simulink model "AION_IDS_SPEEDGOAT"  (R2021a)
settings: configuration reference "AION_IDS_Speedgoat" (kept outside this file)
undefined symbols (not defined in the file): ADCU_SCU_CYCLE_TIME, AutoTrqWhlReq_test, BeamReq_test, BodyCtrlReq_test, BrakeReq_test, C, CONTROL_CYCLE_TIME, GearLvlReq_test, GearLvlReqVD_test, HornRingReq_test, LatCtrlReq_test, LngCtrlReq_test, SCU_ADCU_CYCLE_TIME, SteerAngReq_test, SteerWhlTorqReq_test, TurnLightReq_test
libraries: canmsglib x21, speedgoatlib_IO612 x8, simulink x1
(part 2 of 2)

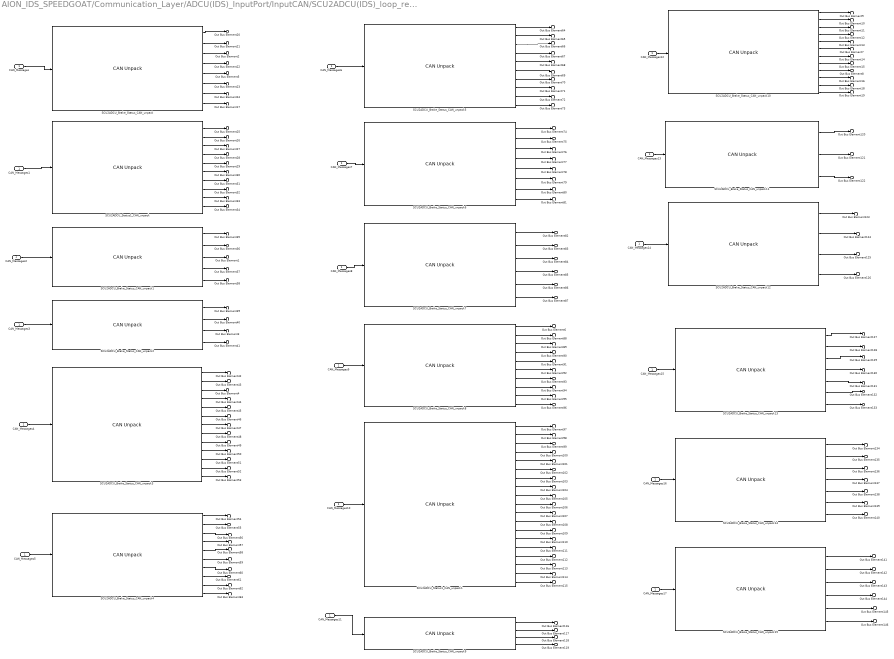
== system AION_IDS_SPEEDGOAT/Communication_Layer/ADCU(IDS)_InputPort/InputCAN/SCU2ADCU(IDS)_loop_receive/CAN_unpack_SCU2ADCU ==
  CAN_Messages : Inport
  CAN_Messages{1..17} (17 alike) : InportShadow
  SCU2ADCU_Brake_Status_CAN_unpack : canmsglib/CAN Unpack  CANdbFile=data\DBC\AION_ADCU_LX_L4_V1.6.1_210531.dbc  MsgList=SCU_1  MsgName=SCU_1  MsgIDType=Standard (11-bit identifier)  MsgIdentifier=384  MsgLength=8  SignalInfo={'BCS_ABSActiveSt','1','1','BE','unsigned','Standard','0','1','0','0','1';'BCS_ABSFaultSt','2','1','BE','unsigned','Standard','0','1','0','0','1';'BCS_VDCActiveSt','53','1','BE','unsigned','Standard','0','1','0','0','1';'BCS_VDCFaultSt','7','1','BE','unsigned','Standard','0','1','0','0','1';'BCS_VehSpd','40','13','BE','unsigned','Standard','0','0.05625','0','0','240';'BCS_VehSpdVD','37','1','BE','unsigned','Standard','0','1','0','0','1';'SCU_1_Checksum','56','8','BE','unsigned','Standard','0','1','0','0','255';'SCU_1_MsgCounter','48','4','BE','unsigned','Standard','0','1','0','0','15'}  IDPort=off  TimestampPort=off  ErrorPort=off  RemotePort=off  LengthPort=off  StatusPort=off  ApplyMinMax=off
      settings: SourceProductBaseCode=ME,XP,VN  DataFormat=CANdb specified signals
  SCU2ADCU_Brake_Status_CAN_unpack1 : canmsglib/CAN Unpack  CANdbFile=data\DBC\AION_ADCU_LX_L4_V1.6.1_210531.dbc  MsgList=SCU_3  MsgName=SCU_3  MsgIDType=Standard (11-bit identifier)  MsgIdentifier=547  MsgLength=8  SignalInfo={'BCS_YawRate','8','12','BE','unsigned','Standard','0','0.00097656','-2.0943','-2.0943','1.9047';'BCS_YawRateOffset','24','12','BE','unsigned','Standard','0','0.00097656','-0.13','-0.13','0.13';'BCS_YawRateSt','4','1','BE','unsigned','Standard','0','1','0','0','1';'SCU_3_Checksum','56','8','BE','unsigned','Standard','0','1','0','0','255';'SCU_3_MsgCounter','20','4','BE','unsigned','Standard','0','1','0','0','15'}  IDPort=off  TimestampPort=off  ErrorPort=off  RemotePort=off  LengthPort=off  StatusPort=off  ApplyMinMax=off
      settings: SourceProductBaseCode=ME,XP,VN  DataFormat=CANdb specified signals
  SCU2ADCU_Brake_Status_CAN_unpack10 : canmsglib/CAN Unpack  CANdbFile=data\DBC\AION_ADCU_LX_L4_V1.6.1_210531.dbc  MsgList=SCU_13  MsgName=SCU_13  MsgIDType=Standard (11-bit identifier)  MsgIdentifier=554  MsgLength=8  SignalInfo={'SCU_13_Checksum','56','8','BE','unsigned','Standard','0','1','0','0','255';'SCU_13_MsgCounter','48','4','BE','unsigned','Standard','0','1','0','0','15';'SCU_EStopSwSt','4','1','BE','unsigned','Standard','0','1','0','0','1';'SCU_EStopSwStVD','5','1','BE','unsigned','Standard','0','1','0','0','1';'SCU_LatAutoCheckReport','52','4','BE','unsigned','Standard','0','1','0','0','15';'SCU_LatCtrlMode','2','2','BE','unsigned','Standard','0','1','0','0','3';'SCU_LatQuitReport','24','8','BE','unsigned','Standard','0','1','0','0','255';'SCU_LngAutoChecklReport','40','16','BE','unsigned','Standard','0','1','0','0','65535';'SCU_LngCtrlMode','0','2','BE','unsigned','Standard','0','1','0','0','3';'SCU_LngQuitReport','16','16','BE','unsigned','Standard','0','1','0','0','65535';'SCU_StrngWhlIntv','7','1','BE','unsigned','Standard','0','1','0','0','1';'VCU_GearLeverIntv','6','1','BE','unsigned','Standard','0','1','0','0','1'}  IDPort=off  TimestampPort=off  ErrorPort=off  RemotePort=off  LengthPort=off  StatusPort=off  ApplyMinMax=off
      settings: SourceProductBaseCode=ME,XP,VN  DataFormat=CANdb specified signals
  SCU2ADCU_Brake_Status_CAN_unpack11 : canmsglib/CAN Unpack  CANdbFile=data\DBC\AION_ADCU_LX_L4_V1.6.1_210531.dbc  MsgList=SCU_14  MsgName=SCU_14  MsgIDType=Standard (11-bit identifier)  MsgIdentifier=706  MsgLength=8  SignalInfo={'VCU_VehDrvMod','11','3','BE','unsigned','Standard','0','1','0','0','7';'VCU_VehRdySt','10','1','BE','unsigned','Standard','0','1','0','0','1';'VCU_VehRng','14','10','BE','unsigned','Standard','0','1','0','0','1000'}  IDPort=off  TimestampPort=off  ErrorPort=off  RemotePort=off  LengthPort=off  StatusPort=off  ApplyMinMax=off
      settings: SourceProductBaseCode=ME,XP,VN  DataFormat=CANdb specified signals
  SCU2ADCU_Brake_Status_CAN_unpack12 : canmsglib/CAN Unpack  CANdbFile=data\DBC\AION_ADCU_LX_L4_V1.6.1_210531.dbc  MsgList=SCU_15  MsgName=SCU_15  MsgIDType=Standard (11-bit identifier)  MsgIdentifier=555  MsgLength=8  SignalInfo={'VCU_ActRecpTorq','16','10','BE','unsigned','Standard','0','2','0','0','2000';'VCU_ActRecpTorqSt','10','2','BE','unsigned','Standard','0','1','0','0','3';'VCU_CrntGearLvl','36','3','BE','unsigned','Standard','0','1','0','0','7';'VCU_CrntGearLvlVD','35','1','BE','unsigned','Standard','0','1','0','0','1'}  IDPort=off  TimestampPort=off  ErrorPort=off  RemotePort=off  LengthPort=off  StatusPort=off  ApplyMinMax=off
      settings: SourceProductBaseCode=ME,XP,VN  DataFormat=CANdb specified signals
  SCU2ADCU_Brake_Status_CAN_unpack13 : canmsglib/CAN Unpack  CANdbFile=data\DBC\AION_ADCU_LX_L4_V1.6.1_210531.dbc  MsgList=SCU_16  MsgName=SCU_16  MsgIDType=Standard (11-bit identifier)  MsgIdentifier=556  MsgLength=8  SignalInfo={'SCU_16_Checksum','56','8','BE','unsigned','Standard','0','1','0','0','205';'SCU_16_MsgCounter','48','4','BE','unsigned','Standard','0','1','0','0','15';'VCU_ACCMaxRecpDecel','16','8','BE','unsigned','Standard','0','0.05','-5','-5','7.75';'VCU_ACCMaxRecpDecelVD','26','1','BE','unsigned','Standard','0','1','0','0','1';'VCU_ActVehWheelTorq','42','14','BE','unsigned','Standard','0','1','0','0','10000';'VCU_LateralAssistBtnInfo','27','1','BE','unsigned','Standard','0','1','0','0','1';'VCU_LateralAssistBtnInfoVD','28','1','BE','unsigned','Standard','0','1','0','0','1'}  IDPort=off  TimestampPort=off  ErrorPort=off  RemotePort=off  LengthPort=off  StatusPort=off  ApplyMinMax=off
      settings: SourceProductBaseCode=ME,XP,VN  DataFormat=CANdb specified signals
  SCU2ADCU_Brake_Status_CAN_unpack14 : canmsglib/CAN Unpack  CANdbFile=data\DBC\AION_ADCU_LX_L4_V1.6.1_210531.dbc  MsgList=SCU_17  MsgName=SCU_17  MsgIDType=Standard (11-bit identifier)  MsgIdentifier=557  MsgLength=8  SignalInfo={'SCU_17_Checksum','56','8','BE','unsigned','Standard','0','1','0','0','255';'SCU_17_MsgCounter','48','4','BE','unsigned','Standard','0','1','0','0','15';'VCU_ACCButtInfo','32','8','BE','unsigned','Standard','0','1','0','0','255';'VCU_AccElecECFail','30','1','BE','unsigned','Standard','0','1','0','0','1';'VCU_GasPedalActPst','40','8','BE','unsigned','Standard','0','0.392','0','0','99.96';'VCU_GasPedalActPstVD','27','1','BE','unsigned','Standard','0','1','0','0','1';'VCU_VehWheelTorqMax','10','14','BE','unsigned','Standard','0','1','0','0','10000'}  IDPort=off  TimestampPort=off  ErrorPort=off  RemotePort=off  LengthPort=off  StatusPort=off  ApplyMinMax=off
      settings: SourceProductBaseCode=ME,XP,VN  DataFormat=CANdb specified signals
  SCU2ADCU_Brake_Status_CAN_unpack15 : canmsglib/CAN Unpack  CANdbFile=data\DBC\AION_ADCU_LX_L4_V1.6.1_210531.dbc  MsgList=SCU_18  MsgName=SCU_18  MsgIDType=Standard (11-bit identifier)  MsgIdentifier=559  MsgLength=8  SignalInfo={'SCU_18_Checksum','56','8','BE','unsigned','Standard','0','1','0','0','255';'SCU_18_MsgCounter','48','4','BE','unsigned','Standard','0','1','0','0','15';'VCU_BrkPedalSt','53','1','BE','unsigned','Standard','0','1','0','0','1';'VCU_BrkPedalStVD','54','1','BE','unsigned','Standard','0','1','0','0','1';'VCU_GasPedalVirtualPst','40','8','BE','unsigned','Standard','0','0.392','0','0','99.96';'VCU_GasPedalVirtualPstVD','55','1','BE','unsigned','Standard','0','1','0','0','1'}  IDPort=off  TimestampPort=off  ErrorPort=off  RemotePort=off  LengthPort=off  StatusPort=off  ApplyMinMax=off
      settings: SourceProductBaseCode=ME,XP,VN  DataFormat=CANdb specified signals
  SCU2ADCU_Brake_Status_CAN_unpack2 : canmsglib/CAN Unpack  CANdbFile=data\DBC\AION_ADCU_LX_L4_V1.6.1_210531.dbc  MsgList=SCU_4  MsgName=SCU_4  MsgIDType=Standard (11-bit identifier)  MsgIdentifier=548  MsgLength=8  SignalInfo={'BCS_HDCCtrlSt','19','2','BE','unsigned','Standard','0','1','0','0','3';'BCS_HDCErrSt','22','1','BE','unsigned','Standard','0','1','0','0','1';'SCU_4_Checksum','56','8','BE','unsigned','Standard','0','1','0','0','255';'SCU_4_MsgCounter','27','4','BE','unsigned','Standard','0','1','0','0','15'}  IDPort=off  TimestampPort=off  ErrorPort=off  RemotePort=off  LengthPort=off  StatusPort=off  ApplyMinMax=off
      settings: SourceProductBaseCode=ME,XP,VN  DataFormat=CANdb specified signals
  SCU2ADCU_Brake_Status_CAN_unpack3 : canmsglib/CAN Unpack  CANdbFile=data\DBC\AION_ADCU_LX_L4_V1.6.1_210531.dbc  MsgList=SCU_5  MsgName=SCU_5  MsgIDType=Standard (11-bit identifier)  MsgIdentifier=385  MsgLength=8  SignalInfo={'BCS_AEBActive','34','1','BE','unsigned','Standard','0','1','0','0','1';'BCS_AEBAvailable','35','1','BE','unsigned','Standard','0','1','0','0','1';'BCS_CDDActive','38','1','BE','unsigned','Standard','0','1','0','0','1';'BCS_CDDAvailable','39','1','BE','unsigned','Standard','0','1','0','0','1';'BCS_CDDFail','47','1','BE','unsigned','Standard','0','1','0','0','1';'BCS_MasterCylinderPr','8','12','BE','unsigned','Standard','0','0.1','0','0','250';'BCS_MasterCylinderPrOffset','24','10','BE','unsigned','Standard','0','0.1','-15','-15','15';'BCS_MasterCylinderPrOffsetVD','7','1','BE','unsigned','Standard','0','1','0','0','1';'BCS_MasterCylinderPrVD','6','1','BE','unsigned','Standard','0','1','0','0','1';'BCS_NoBrakeForce','4','1','BE','unsigned','Standard','0','1','0','0','1';'BCS_VehicleStandStillSt','41','2','BE','unsigned','Standard','0','1','0','0','3';'SCU_5_Checksum','56','8','BE','unsigned','Standard','0','1','0','0','255';'SCU_5_MsgCounter','20','4','BE','unsigned','Standard','0','1','0','0','15'}  IDPort=off  TimestampPort=off  ErrorPort=off  RemotePort=off  LengthPort=off  StatusPort=off  ApplyMinMax=off
      settings: SourceProductBaseCode=ME,XP,VN  DataFormat=CANdb specified signals
  SCU2ADCU_Brake_Status_CAN_unpack4 : canmsglib/CAN Unpack  CANdbFile=data\DBC\AION_ADCU_LX_L4_V1.6.1_210531.dbc  MsgList=SCU_6  MsgName=SCU_6  MsgIDType=Standard (11-bit identifier)  MsgIdentifier=549  MsgLength=8  SignalInfo={'BCS_FLWheelRotatedDirection','6','1','BE','unsigned','Standard','0','1','0','0','1';'BCS_FLWheelRotatedDirectionVD','7','1','BE','unsigned','Standard','0','1','0','0','1';'BCS_FLWheelSpd','16','13','BE','unsigned','Standard','0','0.05625','0','0','240';'BCS_FLWheelSpdVD','5','1','BE','unsigned','Standard','0','1','0','0','1';'BCS_FRWheelRotatedDirection','30','1','BE','unsigned','Standard','0','1','0','0','1';'BCS_FRWheelRotatedDirectionVD','29','1','BE','unsigned','Standard','0','1','0','0','1';'BCS_FRWheelSpd','32','13','BE','unsigned','Standard','0','0.05625','0','0','240';'BCS_FRWheelSpdVD','31','1','BE','unsigned','Standard','0','1','0','0','1';'SCU_6_Checksum','56','8','BE','unsigned','Standard','0','1','0','0','255';'SCU_6_MsgCounter','48','4','BE','unsigned','Standard','0','1','0','0','15'}  IDPort=off  TimestampPort=off  ErrorPort=off  RemotePort=off  LengthPort=off  StatusPort=off  ApplyMinMax=off
      settings: SourceProductBaseCode=ME,XP,VN  DataFormat=CANdb specified signals
  SCU2ADCU_Brake_Status_CAN_unpack5 : canmsglib/CAN Unpack  CANdbFile=data\DBC\AION_ADCU_LX_L4_V1.6.1_210531.dbc  MsgList=SCU_7  MsgName=SCU_7  MsgIDType=Standard (11-bit identifier)  MsgIdentifier=550  MsgLength=8  SignalInfo={'BCS_RLWheelRotatedDirection','6','1','BE','unsigned','Standard','0','1','0','0','1';'BCS_RLWheelRotatedDirectionVD','7','1','BE','unsigned','Standard','0','1','0','0','1';'BCS_RLWheelSpd','16','13','BE','unsigned','Standard','0','0.05625','0','0','240';'BCS_RLWheelSpdVD','5','1','BE','unsigned','Standard','0','1','0','0','1';'BCS_RRWheelRotatedDirection','30','1','BE','unsigned','Standard','0','1','0','0','1';'BCS_RRWheelRotatedDirectionVD','29','1','BE','unsigned','Standard','0','1','0','0','1';'BCS_RRWheelSpd','32','13','BE','unsigned','Standard','0','0.05625','0','0','240';'BCS_RRWheelSpdVD','31','1','BE','unsigned','Standard','0','1','0','0','1';'SCU_7_Checksum','56','8','BE','unsigned','Standard','0','1','0','0','255';'SCU_7_MsgCounter','48','4','BE','unsigned','Standard','0','1','0','0','15'}  IDPort=off  TimestampPort=off  ErrorPort=off  RemotePort=off  LengthPort=off  StatusPort=off  ApplyMinMax=off
      settings: SourceProductBaseCode=ME,XP,VN  DataFormat=CANdb specified signals
  SCU2ADCU_Brake_Status_CAN_unpack6 : canmsglib/CAN Unpack  CANdbFile=data\DBC\AION_ADCU_LX_L4_V1.6.1_210531.dbc  MsgList=SCU_8  MsgName=SCU_8  MsgIDType=Standard (11-bit identifier)  MsgIdentifier=551  MsgLength=8  SignalInfo={'BCS_ActVehLaltrlAccel','36','12','BE','unsigned','Standard','0','0.027127','-21.593','-21.593','21.593';'BCS_ActVehLaltrlAccelVD','53','1','BE','unsigned','Standard','0','1','0','0','1';'BCS_ActVehLongAccel','12','12','BE','unsigned','Standard','0','0.027127','-21.593','-21.593','21.593';'BCS_ActVehLongAccelVD','52','1','BE','unsigned','Standard','0','1','0','0','1';'BCS_VehLaltrlAccelOffset','40','12','BE','unsigned','Standard','0','0.027127','-21.593','-21.593','21.593';'BCS_VehLongAccelOffset','16','12','BE','unsigned','Standard','0','0.027127','-21.593','-21.593','21.593';'SCU_8_Checksum','56','8','BE','unsigned','Standard','0','1','0','0','255';'SCU_8_MsgCounter','48','4','BE','unsigned','Standard','0','1','0','0','15'}  IDPort=off  TimestampPort=off  ErrorPort=off  RemotePort=off  LengthPort=off  StatusPort=off  ApplyMinMax=off
      settings: SourceProductBaseCode=ME,XP,VN  DataFormat=CANdb specified signals
  SCU2ADCU_Brake_Status_CAN_unpack7 : canmsglib/CAN Unpack  CANdbFile=data\DBC\AION_ADCU_LX_L4_V1.6.1_210531.dbc  MsgList=SCU_9  MsgName=SCU_9  MsgIDType=Standard (11-bit identifier)  MsgIdentifier=552  MsgLength=8  SignalInfo={'EPB_FailSt','55','1','BE','unsigned','Standard','0','1','0','0','1';'EPB_SwitchSt','0','2','BE','unsigned','Standard','0','1','0','0','3';'EPB_SwitchStVD','2','1','BE','unsigned','Standard','0','1','0','0','1';'EPB_SysSt','8','3','BE','unsigned','Standard','0','1','0','0','7';'SCU_9_Checksum','56','8','BE','unsigned','Standard','0','1','0','0','255';'SCU_9_MsgCounter','48','4','BE','unsigned','Standard','0','1','0','0','15'}  IDPort=off  TimestampPort=off  ErrorPort=off  RemotePort=off  LengthPort=off  StatusPort=off  ApplyMinMax=off
      settings: SourceProductBaseCode=ME,XP,VN  DataFormat=CANdb specified signals
  SCU2ADCU_Brake_Status_CAN_unpack8 : canmsglib/CAN Unpack  CANdbFile=data\DBC\AION_ADCU_LX_L4_V1.6.1_210531.dbc  MsgList=SCU_10  MsgName=SCU_10  MsgIDType=Standard (11-bit identifier)  MsgIdentifier=553  MsgLength=8  SignalInfo={'EPS_SteeringAngle','16','16','BE','unsigned','Standard','0','0.1','-780','-780','779.9';'EPS_SteeringAngleSpd','38','8','BE','unsigned','Standard','0','4','0','0','1016';'EPS_SteeringAngleSpdVD','7','1','BE','unsigned','Standard','0','1','0','0','1';'EPS_SteeringAngleVD','34','1','BE','unsigned','Standard','0','1','0','0','1';'EPS_StrngWhlTorq','40','8','BE','unsigned','Standard','0','0.1','-12.7','-12.5','12.5';'EPS_StrngWhlTorqVD','0','1','BE','unsigned','Standard','0','1','0','0','1';'EPS_ThermalSt','30','2','BE','unsigned','Standard','0','1','0','0','3';'EPS_WarnLamp','1','1','BE','unsigned','Standard','0','1','0','0','1';'SCU_10_Checksum','56','8','BE','unsigned','Standard','0','1','0','0','255';'SCU_10_MsgCounter','2','4','BE','unsigned','Standard','0','1','0','0','15'}  IDPort=off  TimestampPort=off  ErrorPort=off  RemotePort=off  LengthPort=off  StatusPort=off  ApplyMinMax=off
      settings: SourceProductBaseCode=ME,XP,VN  DataFormat=CANdb specified signals
  SCU2ADCU_Brake_Status_CAN_unpack9 : canmsglib/CAN Unpack  CANdbFile=data\DBC\AION_ADCU_LX_L4_V1.6.1_210531.dbc  MsgList=SCU_12  MsgName=SCU_12  MsgIDType=Standard (11-bit identifier)  MsgIdentifier=705  MsgLength=8  SignalInfo={'SCU_12_Checksum','56','8','BE','unsigned','Standard','0','1','0','0','255';'SCU_12_MsgCounter','48','4','BE','unsigned','Standard','0','1','0','0','15';'SRS_DriverSeatBeltSt','2','2','BE','unsigned','Standard','0','1','0','0','3';'SRS_PsngrSeatBeltSt','0','2','BE','unsigned','Standard','0','1','0','0','3'}  IDPort=off  TimestampPort=off  ErrorPort=off  RemotePort=off  LengthPort=off  StatusPort=off  ApplyMinMax=off
      settings: SourceProductBaseCode=ME,XP,VN  DataFormat=CANdb specified signals
  SCU2ADCU_Status1_CAN_unpack : canmsglib/CAN Unpack  CANdbFile=data\DBC\AION_ADCU_LX_L4_V1.6.1_210531.dbc  MsgList=SCU_2  MsgName=SCU_2  MsgIDType=Standard (11-bit identifier)  MsgIdentifier=546  MsgLength=8  SignalInfo={'BCS_FLWheelSpdEdgesSum','12','12','BE','unsigned','Standard','0','1','0','0','4095';'BCS_FLWheelSpdEdgesSumVD','48','1','BE','unsigned','Standard','0','1','0','0','1';'BCS_FRWheelSpdEdgesSum','16','12','BE','unsigned','Standard','0','1','0','0','4095';'BCS_FRWheelSpdEdgesSumVD','49','1','BE','unsigned','Standard','0','1','0','0','1';'BCS_RLWheelSpdEdgesSum','36','12','BE','unsigned','Standard','0','1','0','0','4095';'BCS_RLWheelSpdEdgesSumVD','50','1','BE','unsigned','Standard','0','1','0','0','1';'BCS_RRWheelSpdEdgesSum','40','12','BE','unsigned','Standard','0','1','0','0','4095';'BCS_RRWheelSpdEdgesSumVD','51','1','BE','unsigned','Standard','0','1','0','0','1';'SCU_2_Checksum','56','8','BE','unsigned','Standard','0','1','0','0','255';'SCU_2_MsgCounter','52','4','BE','unsigned','Standard','0','1','0','0','15'}  IDPort=off  TimestampPort=off  ErrorPort=off  RemotePort=off  LengthPort=off  StatusPort=off  ApplyMinMax=off
      settings: SourceProductBaseCode=ME,XP,VN  DataFormat=CANdb specified signals
  SCU2ADCU_Status1_CAN_unpack1 : canmsglib/CAN Unpack  CANdbFile=data\DBC\AION_ADCU_LX_L4_V1.6.1_210531.dbc  MsgList=SCU_11  MsgName=SCU_11  MsgIDType=Standard (11-bit identifier)  MsgIdentifier=704  MsgLength=8  SignalInfo={'BCM_CtrlAvailable','18','1','BE','unsigned','Standard','0','1','0','0','1';'BCM_DriverDoorAjarSt','8','1','BE','unsigned','Standard','0','1','0','0','1';'BCM_FrontFogLampSt','6','1','BE','unsigned','Standard','0','1','0','0','1';'BCM_FrontWiperSt','0','2','BE','unsigned','Standard','0','1','0','0','3';'BCM_HazardLampSt','16','1','BE','unsigned','Standard','0','1','0','0','1';'BCM_HighBeamSt','5','1','BE','unsigned','Standard','0','1','0','0','1';'BCM_HornSt','17','1','BE','unsigned','Standard','0','1','0','0','1';'BCM_KeySt','2','2','BE','unsigned','Standard','0','1','0','0','3';'BCM_LeftTurnLampFaultSt','13','1','BE','unsigned','Standard','0','1','0','0','1';'BCM_LeftTurnLampSt','12','1','BE','unsigned','Standard','0','1','0','0','1';'BCM_LowBeamSt','4','1','BE','unsigned','Standard','0','1','0','0','1';'BCM_PsngrDoorAjarSt','9','1','BE','unsigned','Standard','0','1','0','0','1';'BCM_RLDoorAjarSt','10','1','BE','unsigned','Standard','0','1','0','0','1';'BCM_RRDoorAjarSt','11','1','BE','unsigned','Standard','0','1','0','0','1';'BCM_RearFogLampSt','7','1','BE','unsigned','Standard','0','1','0','0','1';'BCM_RightTurnLampFaultSt','15','1','BE','unsigned','Standard','0','1','0','0','1';'BCM_RightTurnLampSt','14','1','BE','unsigned','Standard','0','1','0','0','1';'SCU_11_Checksum','56','8','BE','unsigned','Standard','0','1','0','0','255';'SCU_11_MsgCounter','48','4','BE','unsigned','Standard','0','1','0','0','15'}  IDPort=off  TimestampPort=off  ErrorPort=off  RemotePort=off  LengthPort=off  StatusPort=off  ApplyMinMax=off
      settings: SourceProductBaseCode=ME,XP,VN  DataFormat=CANdb specified signals
  Out Bus Element20 : Outport  PortName=SCU2ADCU  Element=SCU_1.BCS_ABSActiveSt
  Out Bus Element21 : Outport  PortName=SCU2ADCU  Element=SCU_1.BCS_ABSFaultSt
  Out Bus Element2 : Outport  PortName=SCU2ADCU  Element=SCU_1.BCS_VDCActiveSt
  Out Bus Element22 : Outport  PortName=SCU2ADCU  Element=SCU_1.BCS_VDCFaultSt
  Out Bus Element5 : Outport  PortName=SCU2ADCU  Element=SCU_1.BCS_VehSpd
  Out Bus Element23 : Outport  PortName=SCU2ADCU  Element=SCU_1.BCS_VehSpdVD
  Out Bus Element24 : Outport  PortName=SCU2ADCU  Element=SCU_1.SCU_1_Checksum
  Out Bus Element17 : Outport  PortName=SCU2ADCU  Element=SCU_1.SCU_1_MsgCounter
  Out Bus Element6 : Outport  PortName=SCU2ADCU  Element=SCU_10.EPS_SteeringAngle
  Out Bus Element88 : Outport  PortName=SCU2ADCU  Element=SCU_10.EPS_SteeringAngleSpd
  Out Bus Element89 : Outport  PortName=SCU2ADCU  Element=SCU_10.EPS_SteeringAngleSpdVD
  Out Bus Element90 : Outport  PortName=SCU2ADCU  Element=SCU_10.EPS_SteeringAngleVD
  Out Bus Element91 : Outport  PortName=SCU2ADCU  Element=SCU_10.EPS_StrngWhlTorq
  Out Bus Element92 : Outport  PortName=SCU2ADCU  Element=SCU_10.EPS_StrngWhlTorqVD
  Out Bus Element93 : Outport  PortName=SCU2ADCU  Element=SCU_10.EPS_ThermalSt
  Out Bus Element94 : Outport  PortName=SCU2ADCU  Element=SCU_10.EPS_WarnLamp
  Out Bus Element95 : Outport  PortName=SCU2ADCU  Element=SCU_10.SCU_10_Checksum
  Out Bus Element96 : Outport  PortName=SCU2ADCU  Element=SCU_10.SCU_10_MsgCounter
  Out Bus Element97 : Outport  PortName=SCU2ADCU  Element=SCU_11.BCM_CtrlAvailable
  Out Bus Element98 : Outport  PortName=SCU2ADCU  Element=SCU_11.BCM_DriverDoorAjarSt
  Out Bus Element99 : Outport  PortName=SCU2ADCU  Element=SCU_11.BCM_FrontFogLampSt
  Out Bus Element100 : Outport  PortName=SCU2ADCU  Element=SCU_11.BCM_FrontWiperSt
  Out Bus Element101 : Outport  PortName=SCU2ADCU  Element=SCU_11.BCM_HazardLampSt
  Out Bus Element102 : Outport  PortName=SCU2ADCU  Element=SCU_11.BCM_HighBeamSt
  Out Bus Element103 : Outport  PortName=SCU2ADCU  Element=SCU_11.BCM_HornSt
  Out Bus Element104 : Outport  PortName=SCU2ADCU  Element=SCU_11.BCM_KeySt
  Out Bus Element105 : Outport  PortName=SCU2ADCU  Element=SCU_11.BCM_LeftTurnLampFaultSt
  Out Bus Element106 : Outport  PortName=SCU2ADCU  Element=SCU_11.BCM_LeftTurnLampSt
  Out Bus Element107 : Outport  PortName=SCU2ADCU  Element=SCU_11.BCM_LowBeamSt
  Out Bus Element108 : Outport  PortName=SCU2ADCU  Element=SCU_11.BCM_PsngrDoorAjarSt
  Out Bus Element109 : Outport  PortName=SCU2ADCU  Element=SCU_11.BCM_RLDoorAjarSt
  Out Bus Element110 : Outport  PortName=SCU2ADCU  Element=SCU_11.BCM_RRDoorAjarSt
  Out Bus Element111 : Outport  PortName=SCU2ADCU  Element=SCU_11.BCM_RearFogLampSt
  Out Bus Element112 : Outport  PortName=SCU2ADCU  Element=SCU_11.BCM_RightTurnLampFaultSt
  Out Bus Element113 : Outport  PortName=SCU2ADCU  Element=SCU_11.BCM_RightTurnLampSt
  Out Bus Element114 : Outport  PortName=SCU2ADCU  Element=SCU_11.SCU_11_Checksum
  Out Bus Element115 : Outport  PortName=SCU2ADCU  Element=SCU_11.SCU_11_MsgCounter
  Out Bus Element116 : Outport  PortName=SCU2ADCU  Element=SCU_12.SCU_12_Checksum
  Out Bus Element117 : Outport  PortName=SCU2ADCU  Element=SCU_12.SCU_12_MsgCounter
  Out Bus Element118 : Outport  PortName=SCU2ADCU  Element=SCU_12.SRS_DriverSeatBeltSt
  Out Bus Element119 : Outport  PortName=SCU2ADCU  Element=SCU_12.SRS_PsngrSeatBeltSt
  Out Bus Element9 : Outport  PortName=SCU2ADCU  Element=SCU_13.SCU_13_Checksum
  Out Bus Element10 : Outport  PortName=SCU2ADCU  Element=SCU_13.SCU_13_MsgCounter
  Out Bus Element11 : Outport  PortName=SCU2ADCU  Element=SCU_13.SCU_EStopSwSt
  Out Bus Element12 : Outport  PortName=SCU2ADCU  Element=SCU_13.SCU_EStopSwStVD
  Out Bus Element13 : Outport  PortName=SCU2ADCU  Element=SCU_13.SCU_LatAutoCheckReport
  Out Bus Element7 : Outport  PortName=SCU2ADCU  Element=SCU_13.SCU_LatCtrlMode
  Out Bus Element14 : Outport  PortName=SCU2ADCU  Element=SCU_13.SCU_LatQuitReport
  Out Bus Element15 : Outport  PortName=SCU2ADCU  Element=SCU_13.SCU_LngAutoChecklReport
  Out Bus Element8 : Outport  PortName=SCU2ADCU  Element=SCU_13.SCU_LngCtrlMode
  Out Bus Element16 : Outport  PortName=SCU2ADCU  Element=SCU_13.SCU_LngQuitReport
  Out Bus Element18 : Outport  PortName=SCU2ADCU  Element=SCU_13.SCU_StrngWhlIntv
  Out Bus Element19 : Outport  PortName=SCU2ADCU  Element=SCU_13.VCU_GearLeverIntv
  Out Bus Element120 : Outport  PortName=SCU2ADCU  Element=SCU_14.VCU_VehDrvMod
  Out Bus Element121 : Outport  PortName=SCU2ADCU  Element=SCU_14.VCU_VehRdySt
  Out Bus Element122 : Outport  PortName=SCU2ADCU  Element=SCU_14.VCU_VehRng
  Out Bus Element123 : Outport  PortName=SCU2ADCU  Element=SCU_15.VCU_ActRecpTorq
  Out Bus Element124 : Outport  PortName=SCU2ADCU  Element=SCU_15.VCU_ActRecpTorqSt
  Out Bus Element125 : Outport  PortName=SCU2ADCU  Element=SCU_15.VCU_CrntGearLvl
  Out Bus Element126 : Outport  PortName=SCU2ADCU  Element=SCU_15.VCU_CrntGearLvlVD
  Out Bus Element127 : Outport  PortName=SCU2ADCU  Element=SCU_16.SCU_16_Checksum
  Out Bus Element128 : Outport  PortName=SCU2ADCU  Element=SCU_16.SCU_16_MsgCounter
  Out Bus Element129 : Outport  PortName=SCU2ADCU  Element=SCU_16.VCU_ACCMaxRecpDecel
  Out Bus Element130 : Outport  PortName=SCU2ADCU  Element=SCU_16.VCU_ACCMaxRecpDecelVD
  Out Bus Element131 : Outport  PortName=SCU2ADCU  Element=SCU_16.VCU_ActVehWheelTorq
  Out Bus Element132 : Outport  PortName=SCU2ADCU  Element=SCU_16.VCU_LateralAssistBtnInfo
  Out Bus Element133 : Outport  PortName=SCU2ADCU  Element=SCU_16.VCU_LateralAssistBtnInfoVD
  Out Bus Element134 : Outport  PortName=SCU2ADCU  Element=SCU_17.SCU_17_Checksum
  Out Bus Element135 : Outport  PortName=SCU2ADCU  Element=SCU_17.SCU_17_MsgCounter
  Out Bus Element136 : Outport  PortName=SCU2ADCU  Element=SCU_17.VCU_ACCButtInfo
  Out Bus Element137 : Outport  PortName=SCU2ADCU  Element=SCU_17.VCU_AccElecECFail
  Out Bus Element138 : Outport  PortName=SCU2ADCU  Element=SCU_17.VCU_GasPedalActPst
  Out Bus Element139 : Outport  PortName=SCU2ADCU  Element=SCU_17.VCU_GasPedalActPstVD
  Out Bus Element140 : Outport  PortName=SCU2ADCU  Element=SCU_17.VCU_VehWheelTorqMax
  Out Bus Element141 : Outport  PortName=SCU2ADCU  Element=SCU_18.SCU_18_Checksum
  Out Bus Element142 : Outport  PortName=SCU2ADCU  Element=SCU_18.SCU_18_MsgCounter
  Out Bus Element143 : Outport  PortName=SCU2ADCU  Element=SCU_18.VCU_BrkPedalSt
  Out Bus Element144 : Outport  PortName=SCU2ADCU  Element=SCU_18.VCU_BrkPedalStVD
  Out Bus Element145 : Outport  PortName=SCU2ADCU  Element=SCU_18.VCU_GasPedalVirtualPst
  Out Bus Element146 : Outport  PortName=SCU2ADCU  Element=SCU_18.VCU_GasPedalVirtualPstVD
  Out Bus Element25 : Outport  PortName=SCU2ADCU  Element=SCU_2.BCS_FLWheelSpdEdgesSum
  Out Bus Element26 : Outport  PortName=SCU2ADCU  Element=SCU_2.BCS_FLWheelSpdEdgesSumVD
  Out Bus Element27 : Outport  PortName=SCU2ADCU  Element=SCU_2.BCS_FRWheelSpdEdgesSum
  Out Bus Element28 : Outport  PortName=SCU2ADCU  Element=SCU_2.BCS_FRWheelSpdEdgesSumVD
  Out Bus Element29 : Outport  PortName=SCU2ADCU  Element=SCU_2.BCS_RLWheelSpdEdgesSum
  Out Bus Element30 : Outport  PortName=SCU2ADCU  Element=SCU_2.BCS_RLWheelSpdEdgesSumVD
  Out Bus Element31 : Outport  PortName=SCU2ADCU  Element=SCU_2.BCS_RRWheelSpdEdgesSum
  Out Bus Element32 : Outport  PortName=SCU2ADCU  Element=SCU_2.BCS_RRWheelSpdEdgesSumVD
  Out Bus Element33 : Outport  PortName=SCU2ADCU  Element=SCU_2.SCU_2_Checksum
  Out Bus Element34 : Outport  PortName=SCU2ADCU  Element=SCU_2.SCU_2_MsgCounter
  Out Bus Element35 : Outport  PortName=SCU2ADCU  Element=SCU_3.BCS_YawRate
  Out Bus Element36 : Outport  PortName=SCU2ADCU  Element=SCU_3.BCS_YawRateOffset
  Out Bus Element1 : Outport  PortName=SCU2ADCU  Element=SCU_3.BCS_YawRateSt
  Out Bus Element37 : Outport  PortName=SCU2ADCU  Element=SCU_3.SCU_3_Checksum
  Out Bus Element38 : Outport  PortName=SCU2ADCU  Element=SCU_3.SCU_3_MsgCounter
  Out Bus Element39 : Outport  PortName=SCU2ADCU  Element=SCU_4.BCS_HDCCtrlSt
  Out Bus Element40 : Outport  PortName=SCU2ADCU  Element=SCU_4.BCS_HDCErrSt
  Out Bus Element3 : Outport  PortName=SCU2ADCU  Element=SCU_4.SCU_4_Checksum
  Out Bus Element41 : Outport  PortName=SCU2ADCU  Element=SCU_4.SCU_4_MsgCounter
  Out Bus Element42 : Outport  PortName=SCU2ADCU  Element=SCU_5.BCS_AEBActive
  Out Bus Element43 : Outport  PortName=SCU2ADCU  Element=SCU_5.BCS_AEBAvailable
  Out Bus Element4 : Outport  PortName=SCU2ADCU  Element=SCU_5.BCS_CDDActive
  Out Bus Element44 : Outport  PortName=SCU2ADCU  Element=SCU_5.BCS_CDDAvailable
  Out Bus Element45 : Outport  PortName=SCU2ADCU  Element=SCU_5.BCS_CDDFail
  Out Bus Element46 : Outport  PortName=SCU2ADCU  Element=SCU_5.BCS_MasterCylinderPr
  Out Bus Element47 : Outport  PortName=SCU2ADCU  Element=SCU_5.BCS_MasterCylinderPrOffset
  Out Bus Element48 : Outport  PortName=SCU2ADCU  Element=SCU_5.BCS_MasterCylinderPrOffsetVD
  Out Bus Element49 : Outport  PortName=SCU2ADCU  Element=SCU_5.BCS_MasterCylinderPrVD
  Out Bus Element50 : Outport  PortName=SCU2ADCU  Element=SCU_5.BCS_NoBrakeForce
  Out Bus Element51 : Outport  PortName=SCU2ADCU  Element=SCU_5.BCS_VehicleStandStillSt
  Out Bus Element52 : Outport  PortName=SCU2ADCU  Element=SCU_5.SCU_5_Checksum
  Out Bus Element53 : Outport  PortName=SCU2ADCU  Element=SCU_5.SCU_5_MsgCounter
  Out Bus Element54 : Outport  PortName=SCU2ADCU  Element=SCU_6.BCS_FLWheelRotatedDirection
  Out Bus Element55 : Outport  PortName=SCU2ADCU  Element=SCU_6.BCS_FLWheelRotatedDirectionVD
  Out Bus Element56 : Outport  PortName=SCU2ADCU  Element=SCU_6.BCS_FLWheelSpd
  Out Bus Element57 : Outport  PortName=SCU2ADCU  Element=SCU_6.BCS_FLWheelSpdVD
  Out Bus Element58 : Outport  PortName=SCU2ADCU  Element=SCU_6.BCS_FRWheelRotatedDirection
  Out Bus Element59 : Outport  PortName=SCU2ADCU  Element=SCU_6.BCS_FRWheelRotatedDirectionVD
  Out Bus Element60 : Outport  PortName=SCU2ADCU  Element=SCU_6.BCS_FRWheelSpd
  Out Bus Element61 : Outport  PortName=SCU2ADCU  Element=SCU_6.BCS_FRWheelSpdVD
  Out Bus Element62 : Outport  PortName=SCU2ADCU  Element=SCU_6.SCU_6_Checksum
  Out Bus Element63 : Outport  PortName=SCU2ADCU  Element=SCU_6.SCU_6_MsgCounter
  Out Bus Element64 : Outport  PortName=SCU2ADCU  Element=SCU_7.BCS_RLWheelRotatedDirection
  Out Bus Element65 : Outport  PortName=SCU2ADCU  Element=SCU_7.BCS_RLWheelRotatedDirectionVD
  Out Bus Element66 : Outport  PortName=SCU2ADCU  Element=SCU_7.BCS_RLWheelSpd
  Out Bus Element67 : Outport  PortName=SCU2ADCU  Element=SCU_7.BCS_RLWheelSpdVD
  Out Bus Element68 : Outport  PortName=SCU2ADCU  Element=SCU_7.BCS_RRWheelRotatedDirection
  Out Bus Element69 : Outport  PortName=SCU2ADCU  Element=SCU_7.BCS_RRWheelRotatedDirectionVD
  Out Bus Element70 : Outport  PortName=SCU2ADCU  Element=SCU_7.BCS_RRWheelSpd
  Out Bus Element71 : Outport  PortName=SCU2ADCU  Element=SCU_7.BCS_RRWheelSpdVD
  Out Bus Element72 : Outport  PortName=SCU2ADCU  Element=SCU_7.SCU_7_Checksum
  Out Bus Element73 : Outport  PortName=SCU2ADCU  Element=SCU_7.SCU_7_MsgCounter
  Out Bus Element74 : Outport  PortName=SCU2ADCU  Element=SCU_8.BCS_ActVehLaltrlAccel
  Out Bus Element75 : Outport  PortName=SCU2ADCU  Element=SCU_8.BCS_ActVehLaltrlAccelVD
  Out Bus Element76 : Outport  PortName=SCU2ADCU  Element=SCU_8.BCS_ActVehLongAccel
  Out Bus Element77 : Outport  PortName=SCU2ADCU  Element=SCU_8.BCS_ActVehLongAccelVD
  Out Bus Element78 : Outport  PortName=SCU2ADCU  Element=SCU_8.BCS_VehLaltrlAccelOffset
  Out Bus Element79 : Outport  PortName=SCU2ADCU  Element=SCU_8.BCS_VehLongAccelOffset
  Out Bus Element80 : Outport  PortName=SCU2ADCU  Element=SCU_8.SCU_8_Checksum
  Out Bus Element81 : Outport  PortName=SCU2ADCU  Element=SCU_8.SCU_8_MsgCounter
  Out Bus Element82 : Outport  PortName=SCU2ADCU  Element=SCU_9.EPB_FailSt
  Out Bus Element83 : Outport  PortName=SCU2ADCU  Element=SCU_9.EPB_SwitchSt
  Out Bus Element84 : Outport  PortName=SCU2ADCU  Element=SCU_9.EPB_SwitchStVD
  Out Bus Element85 : Outport  PortName=SCU2ADCU  Element=SCU_9.EPB_SysSt
  Out Bus Element86 : Outport  PortName=SCU2ADCU  Element=SCU_9.SCU_9_Checksum
  Out Bus Element87 : Outport  PortName=SCU2ADCU  Element=SCU_9.SCU_9_MsgCounter
  wires:
  CAN_Messages/1 -> SCU2ADCU_Brake_Status_CAN_unpack/1
  SCU2ADCU_Brake_Status_CAN_unpack/4 -> Out Bus Element22/1
  SCU2ADCU_Brake_Status_CAN_unpack/1 -> Out Bus Element20/1
  SCU2ADCU_Brake_Status_CAN_unpack/2 -> Out Bus Element21/1
  SCU2ADCU_Brake_Status_CAN_unpack/6 -> Out Bus Element23/1
  SCU2ADCU_Brake_Status_CAN_unpack/7 -> Out Bus Element24/1
  CAN_Messages1/1 -> SCU2ADCU_Status1_CAN_unpack/1
  SCU2ADCU_Status1_CAN_unpack/1 -> Out Bus Element25/1
  SCU2ADCU_Status1_CAN_unpack/2 -> Out Bus Element26/1
  SCU2ADCU_Status1_CAN_unpack/3 -> Out Bus Element27/1
  CAN_Messages2/1 -> SCU2ADCU_Brake_Status_CAN_unpack1/1
  SCU2ADCU_Brake_Status_CAN_unpack1/3 -> Out Bus Element1/1
  SCU2ADCU_Brake_Status_CAN_unpack1/4 -> Out Bus Element37/1
  SCU2ADCU_Brake_Status_CAN_unpack1/1 -> Out Bus Element35/1
  SCU2ADCU_Brake_Status_CAN_unpack1/5 -> Out Bus Element38/1
  CAN_Messages3/1 -> SCU2ADCU_Brake_Status_CAN_unpack2/1
  SCU2ADCU_Brake_Status_CAN_unpack2/3 -> Out Bus Element3/1
  SCU2ADCU_Brake_Status_CAN_unpack2/4 -> Out Bus Element41/1
  SCU2ADCU_Brake_Status_CAN_unpack2/2 -> Out Bus Element40/1
  SCU2ADCU_Brake_Status_CAN_unpack2/1 -> Out Bus Element39/1
  SCU2ADCU_Brake_Status_CAN_unpack3/7 -> Out Bus Element47/1
  CAN_Messages4/1 -> SCU2ADCU_Brake_Status_CAN_unpack3/1
  SCU2ADCU_Brake_Status_CAN_unpack3/3 -> Out Bus Element4/1
  SCU2ADCU_Brake_Status_CAN_unpack3/4 -> Out Bus Element44/1
  SCU2ADCU_Brake_Status_CAN_unpack3/2 -> Out Bus Element43/1
  SCU2ADCU_Brake_Status_CAN_unpack3/1 -> Out Bus Element42/1
  CAN_Messages5/1 -> SCU2ADCU_Brake_Status_CAN_unpack4/1
  CAN_Messages6/1 -> SCU2ADCU_Brake_Status_CAN_unpack5/1
  CAN_Messages7/1 -> SCU2ADCU_Brake_Status_CAN_unpack6/1
  CAN_Messages8/1 -> SCU2ADCU_Brake_Status_CAN_unpack7/1
  SCU2ADCU_Brake_Status_CAN_unpack10/5 -> Out Bus Element13/1
  SCU2ADCU_Brake_Status_CAN_unpack10/4 -> Out Bus Element12/1
  SCU2ADCU_Brake_Status_CAN_unpack10/1 -> Out Bus Element9/1
  CAN_Messages12/1 -> SCU2ADCU_Brake_Status_CAN_unpack10/1
  SCU2ADCU_Brake_Status_CAN_unpack10/2 -> Out Bus Element10/1
  SCU2ADCU_Brake_Status_CAN_unpack10/7 -> Out Bus Element14/1
  CAN_Messages17/1 -> SCU2ADCU_Brake_Status_CAN_unpack15/1
  CAN_Messages13/1 -> SCU2ADCU_Brake_Status_CAN_unpack11/1
  CAN_Messages14/1 -> SCU2ADCU_Brake_Status_CAN_unpack12/1
  CAN_Messages11/1 -> SCU2ADCU_Brake_Status_CAN_unpack9/1
  CAN_Messages15/1 -> SCU2ADCU_Brake_Status_CAN_unpack13/1
  SCU2ADCU_Brake_Status_CAN_unpack10/6 -> Out Bus Element7/1
  CAN_Messages9/1 -> SCU2ADCU_Brake_Status_CAN_unpack8/1
  CAN_Messages16/1 -> SCU2ADCU_Brake_Status_CAN_unpack14/1
  SCU2ADCU_Brake_Status_CAN_unpack10/3 -> Out Bus Element11/1
  CAN_Messages10/1 -> SCU2ADCU_Status1_CAN_unpack1/1
  SCU2ADCU_Brake_Status_CAN_unpack8/1 -> Out Bus Element6/1
  SCU2ADCU_Brake_Status_CAN_unpack/8 -> Out Bus Element17/1
  SCU2ADCU_Status1_CAN_unpack/5 -> Out Bus Element29/1
  SCU2ADCU_Status1_CAN_unpack/9 -> Out Bus Element33/1
  SCU2ADCU_Status1_CAN_unpack/8 -> Out Bus Element32/1
  SCU2ADCU_Status1_CAN_unpack/7 -> Out Bus Element31/1
  SCU2ADCU_Status1_CAN_unpack/6 -> Out Bus Element30/1
  SCU2ADCU_Brake_Status_CAN_unpack3/8 -> Out Bus Element48/1
  SCU2ADCU_Brake_Status_CAN_unpack10/8 -> Out Bus Element15/1
  SCU2ADCU_Brake_Status_CAN_unpack10/11 -> Out Bus Element18/1
  SCU2ADCU_Brake_Status_CAN_unpack10/9 -> Out Bus Element8/1
  SCU2ADCU_Brake_Status_CAN_unpack10/10 -> Out Bus Element16/1
  SCU2ADCU_Brake_Status_CAN_unpack/3 -> Out Bus Element2/1
  SCU2ADCU_Brake_Status_CAN_unpack/5 -> Out Bus Element5/1
  SCU2ADCU_Brake_Status_CAN_unpack10/12 -> Out Bus Element19/1
  SCU2ADCU_Status1_CAN_unpack/4 -> Out Bus Element28/1
  SCU2ADCU_Status1_CAN_unpack/10 -> Out Bus Element34/1
  SCU2ADCU_Brake_Status_CAN_unpack1/2 -> Out Bus Element36/1
  SCU2ADCU_Brake_Status_CAN_unpack3/5 -> Out Bus Element45/1
  SCU2ADCU_Brake_Status_CAN_unpack3/6 -> Out Bus Element46/1
  SCU2ADCU_Brake_Status_CAN_unpack3/9 -> Out Bus Element49/1
  SCU2ADCU_Brake_Status_CAN_unpack3/10 -> Out Bus Element50/1
  SCU2ADCU_Brake_Status_CAN_unpack3/11 -> Out Bus Element51/1
  SCU2ADCU_Brake_Status_CAN_unpack3/12 -> Out Bus Element52/1
  SCU2ADCU_Brake_Status_CAN_unpack3/13 -> Out Bus Element53/1
  SCU2ADCU_Brake_Status_CAN_unpack4/1 -> Out Bus Element54/1
  SCU2ADCU_Brake_Status_CAN_unpack4/2 -> Out Bus Element55/1
  SCU2ADCU_Brake_Status_CAN_unpack4/3 -> Out Bus Element56/1
  SCU2ADCU_Brake_Status_CAN_unpack4/4 -> Out Bus Element57/1
  SCU2ADCU_Brake_Status_CAN_unpack4/5 -> Out Bus Element58/1
  SCU2ADCU_Brake_Status_CAN_unpack4/6 -> Out Bus Element59/1
  SCU2ADCU_Brake_Status_CAN_unpack4/7 -> Out Bus Element60/1
  SCU2ADCU_Brake_Status_CAN_unpack4/8 -> Out Bus Element61/1
  SCU2ADCU_Brake_Status_CAN_unpack4/9 -> Out Bus Element62/1
  SCU2ADCU_Brake_Status_CAN_unpack4/10 -> Out Bus Element63/1
  SCU2ADCU_Brake_Status_CAN_unpack5/1 -> Out Bus Element64/1
  SCU2ADCU_Brake_Status_CAN_unpack5/2 -> Out Bus Element65/1
  SCU2ADCU_Brake_Status_CAN_unpack5/3 -> Out Bus Element66/1
  SCU2ADCU_Brake_Status_CAN_unpack5/5 -> Out Bus Element68/1
  SCU2ADCU_Brake_Status_CAN_unpack5/7 -> Out Bus Element70/1
  SCU2ADCU_Brake_Status_CAN_unpack5/8 -> Out Bus Element71/1
  SCU2ADCU_Brake_Status_CAN_unpack5/9 -> Out Bus Element72/1
  SCU2ADCU_Brake_Status_CAN_unpack5/10 -> Out Bus Element73/1
  SCU2ADCU_Brake_Status_CAN_unpack5/4 -> Out Bus Element67/1
  SCU2ADCU_Brake_Status_CAN_unpack5/6 -> Out Bus Element69/1
  SCU2ADCU_Brake_Status_CAN_unpack6/1 -> Out Bus Element74/1
  SCU2ADCU_Brake_Status_CAN_unpack6/2 -> Out Bus Element75/1
  SCU2ADCU_Brake_Status_CAN_unpack6/3 -> Out Bus Element76/1
  SCU2ADCU_Brake_Status_CAN_unpack6/4 -> Out Bus Element77/1
  SCU2ADCU_Brake_Status_CAN_unpack6/5 -> Out Bus Element78/1
  SCU2ADCU_Brake_Status_CAN_unpack6/6 -> Out Bus Element79/1
  SCU2ADCU_Brake_Status_CAN_unpack6/7 -> Out Bus Element80/1
  SCU2ADCU_Brake_Status_CAN_unpack6/8 -> Out Bus Element81/1
  SCU2ADCU_Brake_Status_CAN_unpack7/1 -> Out Bus Element82/1
  SCU2ADCU_Brake_Status_CAN_unpack7/2 -> Out Bus Element83/1
  SCU2ADCU_Brake_Status_CAN_unpack7/3 -> Out Bus Element84/1
  SCU2ADCU_Brake_Status_CAN_unpack7/4 -> Out Bus Element85/1
  SCU2ADCU_Brake_Status_CAN_unpack7/5 -> Out Bus Element86/1
  SCU2ADCU_Brake_Status_CAN_unpack7/6 -> Out Bus Element87/1
  SCU2ADCU_Brake_Status_CAN_unpack8/10 -> Out Bus Element96/1
  SCU2ADCU_Brake_Status_CAN_unpack8/2 -> Out Bus Element88/1
  SCU2ADCU_Brake_Status_CAN_unpack8/3 -> Out Bus Element89/1
  SCU2ADCU_Brake_Status_CAN_unpack8/4 -> Out Bus Element90/1
  SCU2ADCU_Brake_Status_CAN_unpack8/5 -> Out Bus Element91/1
  SCU2ADCU_Brake_Status_CAN_unpack8/6 -> Out Bus Element92/1
  SCU2ADCU_Brake_Status_CAN_unpack8/7 -> Out Bus Element93/1
  SCU2ADCU_Brake_Status_CAN_unpack8/8 -> Out Bus Element94/1
  SCU2ADCU_Brake_Status_CAN_unpack8/9 -> Out Bus Element95/1
  SCU2ADCU_Status1_CAN_unpack1/1 -> Out Bus Element97/1
  SCU2ADCU_Status1_CAN_unpack1/2 -> Out Bus Element98/1
  SCU2ADCU_Status1_CAN_unpack1/3 -> Out Bus Element99/1
  SCU2ADCU_Status1_CAN_unpack1/4 -> Out Bus Element100/1
  SCU2ADCU_Status1_CAN_unpack1/5 -> Out Bus Element101/1
  SCU2ADCU_Status1_CAN_unpack1/6 -> Out Bus Element102/1
  SCU2ADCU_Status1_CAN_unpack1/7 -> Out Bus Element103/1
  SCU2ADCU_Status1_CAN_unpack1/8 -> Out Bus Element104/1
  SCU2ADCU_Status1_CAN_unpack1/9 -> Out Bus Element105/1
  SCU2ADCU_Status1_CAN_unpack1/10 -> Out Bus Element106/1
  SCU2ADCU_Status1_CAN_unpack1/11 -> Out Bus Element107/1
  SCU2ADCU_Status1_CAN_unpack1/12 -> Out Bus Element108/1
  SCU2ADCU_Status1_CAN_unpack1/13 -> Out Bus Element109/1
  SCU2ADCU_Status1_CAN_unpack1/14 -> Out Bus Element110/1
  SCU2ADCU_Status1_CAN_unpack1/15 -> Out Bus Element111/1
  SCU2ADCU_Status1_CAN_unpack1/16 -> Out Bus Element112/1
  SCU2ADCU_Status1_CAN_unpack1/17 -> Out Bus Element113/1
  SCU2ADCU_Status1_CAN_unpack1/18 -> Out Bus Element114/1
  SCU2ADCU_Status1_CAN_unpack1/19 -> Out Bus Element115/1
  SCU2ADCU_Brake_Status_CAN_unpack9/3 -> Out Bus Element118/1
  SCU2ADCU_Brake_Status_CAN_unpack9/1 -> Out Bus Element116/1
  SCU2ADCU_Brake_Status_CAN_unpack9/2 -> Out Bus Element117/1
  SCU2ADCU_Brake_Status_CAN_unpack9/4 -> Out Bus Element119/1
  SCU2ADCU_Brake_Status_CAN_unpack11/2 -> Out Bus Element121/1
  SCU2ADCU_Brake_Status_CAN_unpack11/1 -> Out Bus Element120/1
  SCU2ADCU_Brake_Status_CAN_unpack11/3 -> Out Bus Element122/1
  SCU2ADCU_Brake_Status_CAN_unpack12/1 -> Out Bus Element123/1
  SCU2ADCU_Brake_Status_CAN_unpack12/2 -> Out Bus Element124/1
  SCU2ADCU_Brake_Status_CAN_unpack12/3 -> Out Bus Element125/1
  SCU2ADCU_Brake_Status_CAN_unpack12/4 -> Out Bus Element126/1
  SCU2ADCU_Brake_Status_CAN_unpack13/2 -> Out Bus Element128/1
  SCU2ADCU_Brake_Status_CAN_unpack13/4 -> Out Bus Element130/1
  SCU2ADCU_Brake_Status_CAN_unpack13/7 -> Out Bus Element133/1
  SCU2ADCU_Brake_Status_CAN_unpack13/1 -> Out Bus Element127/1
  SCU2ADCU_Brake_Status_CAN_unpack13/3 -> Out Bus Element129/1
  SCU2ADCU_Brake_Status_CAN_unpack13/5 -> Out Bus Element131/1
  SCU2ADCU_Brake_Status_CAN_unpack13/6 -> Out Bus Element132/1
  SCU2ADCU_Brake_Status_CAN_unpack14/1 -> Out Bus Element134/1
  SCU2ADCU_Brake_Status_CAN_unpack14/4 -> Out Bus Element137/1
  SCU2ADCU_Brake_Status_CAN_unpack14/5 -> Out Bus Element138/1
  SCU2ADCU_Brake_Status_CAN_unpack14/6 -> Out Bus Element139/1
  SCU2ADCU_Brake_Status_CAN_unpack14/7 -> Out Bus Element140/1
  SCU2ADCU_Brake_Status_CAN_unpack14/2 -> Out Bus Element135/1
  SCU2ADCU_Brake_Status_CAN_unpack14/3 -> Out Bus Element136/1
  SCU2ADCU_Brake_Status_CAN_unpack15/1 -> Out Bus Element141/1
  SCU2ADCU_Brake_Status_CAN_unpack15/4 -> Out Bus Element144/1
  SCU2ADCU_Brake_Status_CAN_unpack15/2 -> Out Bus Element142/1
  SCU2ADCU_Brake_Status_CAN_unpack15/5 -> Out Bus Element145/1
  SCU2ADCU_Brake_Status_CAN_unpack15/6 -> Out Bus Element146/1
  SCU2ADCU_Brake_Status_CAN_unpack15/3 -> Out Bus Element143/1

== matlab function AION_IDS_SPEEDGOAT/Application_Layer/Signal_test/Subsystem2/MATLAB Function ==
  data: u input; get_VehRdySt output
function get_VehRdySt = fcn(u)

get_VehRdySt = u;
end

== matlab function AION_IDS_SPEEDGOAT/Application_Layer/Signal_test/Subsystem2/MATLAB Function2 ==
  data: u input; get_LatCtrlMode output
function get_LatCtrlMode = fcn(u)

get_LatCtrlMode = u;
end

== matlab function AION_IDS_SPEEDGOAT/Application_Layer/Signal_test/Subsystem2/MATLAB Function3 ==
  data: u input; get_SteeringAngle output
function get_SteeringAngle = fcn(u)

get_SteeringAngle = u;
end

== matlab function AION_IDS_SPEEDGOAT/Application_Layer/Signal_test/Subsystem2/MATLAB Function4 ==
  data: u input; get_LngCtrlMode output
function get_LngCtrlMode = fcn(u)

get_LngCtrlMode = u;
end

== matlab function AION_IDS_SPEEDGOAT/Application_Layer/Signal_test/Subsystem2/MATLAB Function5 ==
  data: u input; get_CrntGearLvl output
function get_CrntGearLvl = fcn(u)

get_CrntGearLvl = u;
end

== matlab function AION_IDS_SPEEDGOAT/Application_Layer/Signal_test/Subsystem2/MATLAB Function6 ==
  data: u input; get_VehSpd output
function get_VehSpd = fcn(u)

get_VehSpd = u;
end

== matlab function AION_IDS_SPEEDGOAT/Application_Layer/Signal_test/Subsystem2/MATLAB Function7 ==
  data: u input; get_CtrlAvailable output
function get_CtrlAvailable = fcn(u)

get_CtrlAvailable = u;
end

== matlab function AION_IDS_SPEEDGOAT/Application_Layer/Signal_test/Subsystem2/MATLAB Function8 ==
  data: u input; get_HazardLampSt output
function get_HazardLampSt = fcn(u)

get_HazardLampSt = u;
end

== matlab function AION_IDS_SPEEDGOAT/Application_Layer/Signal_test/Subsystem2/MATLAB Function1 ==
  data: u input; get_VehDrvMod output
function get_VehDrvMod = fcn(u)

get_VehDrvMod = u;
end

== matlab function AION_IDS_SPEEDGOAT/Application_Layer/Signal_test/Subsystem2/MATLAB Function9 ==
  data: u input; get_HornSt output
function get_HornSt = fcn(u)

get_HornSt = u;
end

== matlab function AION_IDS_SPEEDGOAT/Application_Layer/Signal_test/Subsystem2/MATLAB Function10 ==
  data: u input; get_LowBeamSt output
function get_LowBeamSt = fcn(u)

get_LowBeamSt = u;
end

== matlab function AION_IDS_SPEEDGOAT/Application_Layer/Signal_test/Subsystem2/MATLAB Function11 ==
  data: u input; get_HighBeamSt output
function get_HighBeamSt = fcn(u)

get_HighBeamSt = u;
end

== matlab function AION_IDS_SPEEDGOAT/Application_Layer/Signal_test/Subsystem2/MATLAB Function12 ==
  data: u input; get_LeftTurnLampSt output
function get_LeftTurnLampSt = fcn(u)

get_LeftTurnLampSt = u;
end

== matlab function AION_IDS_SPEEDGOAT/Application_Layer/Signal_test/Subsystem2/MATLAB Function13 ==
  data: u input; get_RightTurnLampSt output
function get_RightTurnLampSt = fcn(u)

get_RightTurnLampSt = u;
end
